simulink model "Bowwave2Drogue_v6_addControl_VR_tkTur2"  (R2013a)
settings: Solver=ode4  StartTime=0.0  StopTime=50  FixedStep=0.02  RelTol=1e-5  AbsTol=1e-4
InitFcn:
  | F16InitData_slow
values from neighbouring files (symbols this model uses):
  A_full = [ ... (first row only)    [F16InitData.m]    (also in F16InitData_slow.m)
  B_full = [ ... (first row only)    [F16InitData.m]    (also in F16InitData_slow.m)
  B_wTur = zeros(12,6)    [F16InitData.m]    (also in F16InitData_slow.m = A_full*Csta*Cb_e; F16_2003hiModelAutopilot.m = A*Csta*Cb_e)
  C_attitude = [0 0 0 1 0 0 0 0 0 0 0 0 ... (first row only)    [F16InitData.m]    (also in F16InitData_slow.m; F16_2003hiModelAutopilot.m = [zeros(3,3),eye(3),zeros(3,12)])
  C_xd_h_yd = [ ... (first row only)    [F16InitData.m]    (also in F16InitData_slow.m)
  C_xd_h_yd2m = [C_xd_h_yd2m(1,:) ... (first row only)    [F16InitData.m]    (also in F16InitData_slow.m)
  Kc = diag([0.3048,0.3048,0.3048,rad2degree,rad2degree,rad2degree,1,0.3048,rad2degree,rad2degree,rad2degree,rad2degree])    [F16InitData.m]    (also in F16InitData1.m = [1	0	0	0	0	0	0	0	0	0	0	0	0	0	0	0	0	0; F16InitData_slow.m; F16_2003hiModelAutopilot.m = [)
  Ki = [ ... (first row only)    [F16InitData.m]    (also in F16InitData_slow.m = [1.97872869	0.650510465	0; F16_2003hiModelAutopilot.m = zeros(4,3))
  Kp = [ ... (first row only)    [F16InitData.m]    (also in F16InitData_slow.m; F16_2003hiModelAutopilot.m = zeros(4,18))
  m2ft = 1/0.3048    (= 3.28083989501)    [F16InitData.m]    (also in F16InitData_slow.m; F16_2003hiModelAutopilot.m)
  q = zeros(N,1)    [hose3D_n_air_Fv_correction.m]
  trim_control = [-3.132 ... (first row only)    [F16InitData.m]    (also in F16InitData1.m = [-1.549425813; F16InitData_slow.m; F16_2003hiModelAutopilot.m = [-2.979731649)
  trim_state = [ ... (first row only)    [F16InitData.m]    (also in F16InitData1.m = [0; F16InitData_slow.m; F16_2003hiModelAutopilot.m)
  trim_thrust = 0.17766    [F16InitData.m]    (also in F16InitData1.m = -206727.459732; F16InitData_slow.m; F16NolinearModelInitialData.m = 5000; F16_2003hiModelAutopilot.m = 2279.08519955)
  X1_0 = [0 0 0 0 0 0 0 0 0 0 0 0]'    [F16InitData.m]    (also in F16InitData1.m = zeros(18,1); F16InitData_slow.m; F16_2003hiModelAutopilot.m = zeros(18,1))
undefined symbols (not defined in the file or in its folder): F, Light, MIL
libraries: simulink x5, aerolibwind2 x3, vrlib x1
settings Model: Creator=WhisPer  LastModifiedBy=Dai

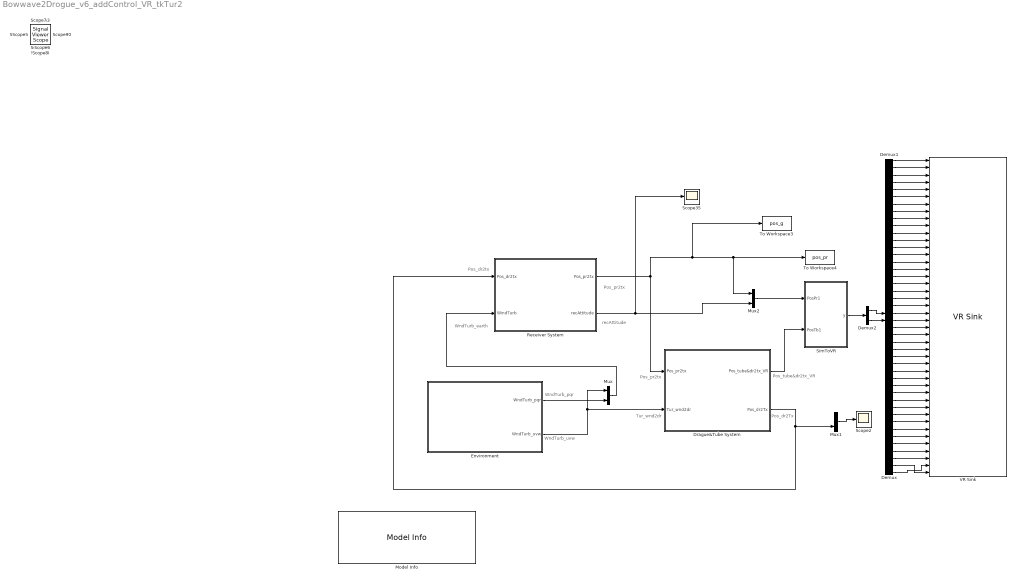
== system Bowwave2Drogue_v6_addControl_VR_tkTur2 ==
  note: recAttitude
  note: WndTurb_uvw
  note: WndTurb_pqr
  note: Pos_dr2Tx
  note: Pos_tube&dr2tx_VR
  note: Tur_wnd2dr
  note: Pos_pr2tx
  note: WndTurb_earth
  note: Pos_dr2tx
  note: Pos_pr2tx
  Demux : Demux  Outputs=22
  Demux1 : Demux  Outputs=22
  Demux2 : Demux  Outputs=[88,66]
  Drague&Tube System : Subsystem
      mask Display: image(imread('Icon\zhuitao.png'))
  Environment : Subsystem
      mask Display: image(imread('Icon\Enviroment.jpg'))
  Model Info : simulink/Model-Wide Utilities/Model Info  InitialBlockCM=None  BlockCM=None  Frame=on  DisplayStringWithTags=|  HorizontalTextAlignment=Center  LeftAlignmentValue=0.5  SourceBlockDiagram=Bowwave2Drogue_v6_addControl_VR_tkTur2  TagMaxNumber=20
      | Ppr_rc=[6.06 0.54 -0.86]
      | Pns_rc=[8.00 0.00  0.00]
      | Pfl_rc=[3.75 0.00 -0.86]
      | Pdr0_tk=[-13.549 0.00 5]
  Mux : Mux  Inputs=2
  Mux1 : Mux  Inputs=2
  Mux2 : Mux  Inputs=2
  Receiver System : Subsystem
      mask Display: image(imread('Icon\f16thumb.jpg'))
  Scope2 : Scope
      settings: YMin=-22.5  YMax=7.5  SaveName=ScopeData18
  Scope35 : Scope
      settings: YMin=-0.225  YMax=0.15  SaveName=ScopeData19
  SimToVR : MATLAB Function  TreatAsAtomicUnit=on
  To Workspace3 : ToWorkspace  VariableName=pos_g  SampleTime=-1
  To Workspace4 : ToWorkspace  VariableName=pos_pr  SampleTime=-1
  VR Sink : vrlib/VR Sink  InstantiateOnLoad=on  SampleTime=-1  ViewEnable=on  RemoteChange=off  RemoteView=off  FieldsWritten=tube1.rotation.4.1.1.double#tube1.translation.3.1.1.double#tube2.rotation.4.1.1.double#tube2.translation.3.1.1.double#tube3.rotation.4.1.1.double#tube3.translation.3.1.1.double#tube4.rotation.4.1.1.double#tube4.translation.3.1.1.double#tube5.rotation.4.1.1.double#tube5.translation.3.1.1.double#tube6.rotation.4.1.1.double#tube6.translation.3.1.1.double#tube7.rotation.4.1.1.double#tube7.translation.3.1.1.double#tube8.rotation.4.1.1.double#tube8.translation.3.1.1.double#tube9.rotation.4.1.1.double#tube9.translation.3.1.1.double#tube10.rotation.4.1.1.double#tube10.translation.3.1.1.double#tube11.rotation.4.1.1.double#tube11.translation.3.1.1.double#tube12.rotation.4.1.1.double#tube12.translation.3.1.1.double#tube13.rotation.4.1.1.double#tube13.translation.3.1.1.double#tube14.rotation.4.1.1.double#tube14.translation.3.1.1.double#tube15.rotation.4.1.1.double#tube15.translation.3.1.1.double#tube16.rotation.4.1.1.double#tube16.translation.3.1.1.double#tube17.rotation.4.1.1.double#tube17.translation.3.1.1.double#tube18.rotation.4.1.1.double#tube18.translation.3.1.1.double#tube19.rotation.4.1.1.double#tube19.translation.3.1.1.double#tube20.rotation.4.1.1.double#tube20.translation.3.1.1.double#tube21.rotation.4.1.1.double#tube21.translation.3.1.1.double#ASDD.translation.3.1.1.double#Receiver.rotation.4.1.1.double  WorldFileName=AirRefuelingTubeSim.WRL  AutoView=off  VideoDimensions=[]  AllowVariableSize=off
  Scope{,1,3,5..9,11,13,15..34} (30 alike) : SignalViewerScope  IOType=viewer  RefreshTime=0.035000
      Scope settings: SaveName=ScopeData32
      Scope1 settings: YMin=-40  YMax=15  SaveName=ScopeData33
      Scope11 settings: SaveName=ScopeData7
      Scope13 settings: SaveName=ScopeData10
      Scope15 settings: SaveName=ScopeData12
      Scope16 settings: SaveName=ScopeData13
      Scope17 settings: SaveName=ScopeData14
      Scope18 settings: SaveName=ScopeData15
      Scope19 settings: SaveName=ScopeData16
      Scope20 settings: SaveName=ScopeData17
      Scope21 settings: SaveName=ScopeData18
      Scope22 settings: SaveName=ScopeData19
      Scope23 settings: SaveName=ScopeData20
      Scope24 settings: SaveName=ScopeData21
      Scope25 settings: SaveName=ScopeData22
      Scope26 settings: SaveName=ScopeData23
      Scope27 settings: SaveName=ScopeData24
      Scope28 settings: SaveName=ScopeData25
      Scope29 settings: SaveName=ScopeData26
      Scope3 settings: TimeRange=8  YMin=-2895.619158878505  YMax=-1095.619158878505
      Scope30 settings: SaveName=ScopeData27
      Scope31 settings: SaveName=ScopeData28
      Scope32 settings: SaveName=ScopeData29
      Scope33 settings: SaveName=ScopeData30
      Scope34 settings: YMin=-0.5  YMax=0.9  SaveName=ScopeData31
      Scope5 settings: SaveName=ScopeData2
      Scope6 settings: SaveName=ScopeData3
      Scope7 settings: SaveName=ScopeData4
      Scope8 settings: SaveName=ScopeData5
      Scope9 settings: SaveName=ScopeData9
  Scope10 : SignalViewerScope  IOType=viewer  ZoomMode=yonly  RefreshTime=0.035000
      settings: SaveName=ScopeData6
  Scope12 : SignalViewerScope  IOType=viewer  ZoomMode=xonly  RefreshTime=0.035000
      settings: SaveName=ScopeData8
  Scope14 : SignalViewerScope  IOType=viewer  ZoomMode=yonly  RefreshTime=0.035000
      settings: YMin=-1  YMax=1  SaveName=ScopeData11
  Scope4 : SignalViewerScope  IOType=viewer  ZoomMode=xonly  RefreshTime=0.035000
  wires:
  Receiver System/1(Pos_pr2tx) -> Drague&Tube System/1(Pos_pr2tx), Mux2/1, To Workspace4/1, To Workspace3/1
  Demux2/1 -> Demux1/1
  Demux2/2 -> Demux/1
  SimToVR/1(y) -> Demux2/1
  Drague&Tube System/1(Pos_tube&dr2tx_VR) -> SimToVR/2(PosTb1)
  Drague&Tube System/2(Pos_dr2Tx) -> Receiver System/1(Pos_dr2tx), Mux1/2
  Mux/1 -> Receiver System/2(WindTurb)
  Environment/2(WndTurb_uvw) -> Drague&Tube System/2(Tur_wnd2dr), Mux/1
  Environment/1(WndTurb_pqr) -> Mux/2
  Mux1/1 -> Scope2/1
  Receiver System/2(recAttitude) -> Scope35/1, Mux2/2
  Mux2/1 -> SimToVR/1(PosPr1)
  Demux1/1 -> VR Sink/1
  Demux/1 -> VR Sink/2
  Demux1/2 -> VR Sink/3
  Demux/2 -> VR Sink/4
  Demux1/3 -> VR Sink/5
  Demux/3 -> VR Sink/6
  Demux1/4 -> VR Sink/7
  Demux/4 -> VR Sink/8
  Demux1/5 -> VR Sink/9
  Demux/5 -> VR Sink/10
  Demux1/6 -> VR Sink/11
  Demux/6 -> VR Sink/12
  Demux1/7 -> VR Sink/13
  Demux/7 -> VR Sink/14
  Demux1/8 -> VR Sink/15
  Demux/8 -> VR Sink/16
  Demux1/9 -> VR Sink/17
  Demux/9 -> VR Sink/18
  Demux1/10 -> VR Sink/19
  Demux/10 -> VR Sink/20
  Demux1/11 -> VR Sink/21
  Demux/11 -> VR Sink/22
  Demux1/12 -> VR Sink/23
  Demux/12 -> VR Sink/24
  Demux1/13 -> VR Sink/25
  Demux/13 -> VR Sink/26
  Demux1/14 -> VR Sink/27
  Demux/14 -> VR Sink/28
  Demux1/15 -> VR Sink/29
  Demux/15 -> VR Sink/30
  Demux1/16 -> VR Sink/31
  Demux/16 -> VR Sink/32
  Demux1/17 -> VR Sink/33
  Demux/17 -> VR Sink/34
  Demux1/18 -> VR Sink/35
  Demux/18 -> VR Sink/36
  Demux1/19 -> VR Sink/37
  Demux/19 -> VR Sink/38
  Demux1/20 -> VR Sink/39
  Demux/20 -> VR Sink/40
  Demux1/21 -> VR Sink/41
  Demux/21 -> VR Sink/42
  Demux/22 -> VR Sink/43
  Demux1/22 -> VR Sink/44

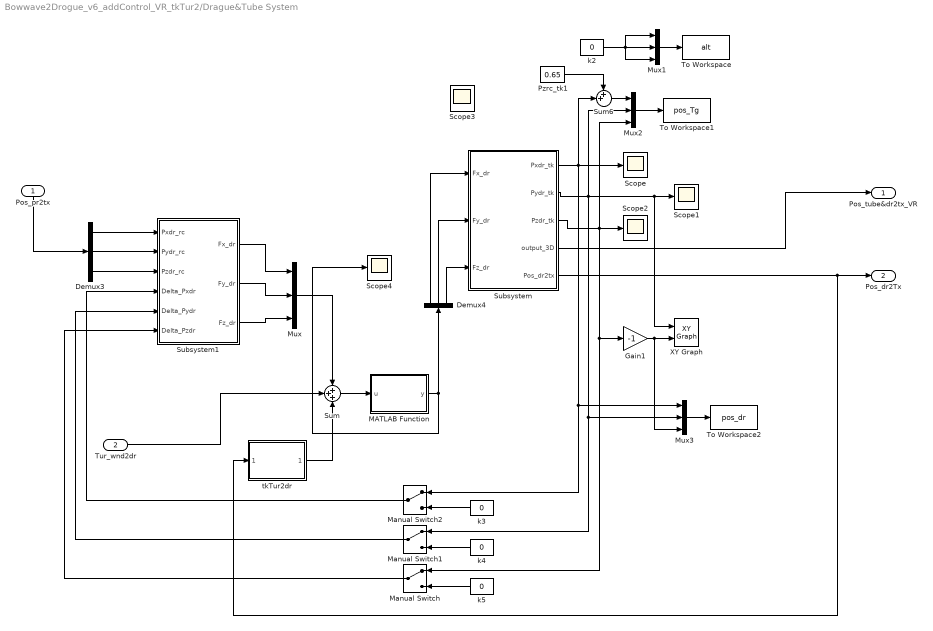
== system Bowwave2Drogue_v6_addControl_VR_tkTur2/Drague&Tube System ==
  Pos_pr2tx : Inport
  Tur_wnd2dr : Inport  Port=2
  Demux3 : Demux  Outputs=3
  Demux4 : Demux  Outputs=3
  Gain1 : Gain  Gain=-1
  MATLAB Function : MATLAB Function  TreatAsAtomicUnit=on
  Manual Switch : ManualSwitch
  Manual Switch1 : ManualSwitch
  Manual Switch2 : ManualSwitch
  Mux{,1..3} (4 alike) : Mux  Inputs=3
  Pzrc_tk1 : Constant  Value=0.65
  Scope{,1..4} (5 alike) : Scope
      Scope1 settings: YMin=-1  YMax=1
      Scope2 settings: SaveName=ScopeData2
      Scope3 settings: YMin=-15.5  YMax=-9  SaveName=ScopeData17
      Scope4 settings: TimeRange=50  YMin=-60  SaveName=ScopeData20
  Subsystem : Subsystem
  Subsystem1 : Subsystem
  Sum : Sum  Inputs=+++
  Sum6 : Sum  Inputs=++|
  To Workspace : ToWorkspace  VariableName=alt  SampleTime=-1
  To Workspace1 : ToWorkspace  VariableName=pos_Tg  SampleTime=-1
  To Workspace2 : ToWorkspace  VariableName=pos_dr  SampleTime=-1
  XY Graph : simulink/Sinks/XY Graph  xmin=-1  xmax=1  ymin=-1-4.65  ymax=1-4.65  st=-1
  k{2..5} (4 alike) : Constant  Value=0
  tkTur2dr : MATLAB Function  TreatAsAtomicUnit=on
  Pos_tube&dr2tx_VR : Outport
  Pos_dr2Tx : Outport  Port=2
  wires:
  Demux3/2 -> Subsystem1/2(Pydr_rc)
  Demux3/3 -> Subsystem1/3(Pzdr_rc)
  Subsystem/5(Pos_dr2tx) -> tkTur2dr/1(pos_dr2tk), Pos_dr2Tx/1
  Subsystem/3(Pzdr_tk) -> Manual Switch/1, Gain1/1, Mux2/3, Scope2/1
  Gain1/1 -> Mux3/3, XY Graph/2
  Subsystem/1(Pxdr_tk) -> Mux3/1, Manual Switch2/1, Scope/1, Sum6/2
  Subsystem/2(Pydr_tk) -> Mux3/2, Manual Switch1/1, Mux2/2, XY Graph/1, Scope1/1
  Manual Switch/1 -> Subsystem1/6(Delta_Pzdr)
  Mux2/1 -> To Workspace1/1
  Mux1/1 -> To Workspace/1
  Mux3/1 -> To Workspace2/1
  k3/1 -> Manual Switch2/2
  k5/1 -> Manual Switch/2
  Pzrc_tk1/1 -> Sum6/1
  k2/1 -> Mux1/3, Mux1/1, Mux1/2
  Sum6/1 -> Mux2/1
  Manual Switch2/1 -> Subsystem1/4(Delta_Pxdr)
  Manual Switch1/1 -> Subsystem1/5(Delta_Pydr)
  k4/1 -> Manual Switch1/2
  Subsystem/4(output_3D) -> Pos_tube&dr2tx_VR/1
  MATLAB Function/1(y) -> Demux4/1, Scope4/1
  Pos_pr2tx/1 -> Demux3/1
  Demux3/1 -> Subsystem1/1(Pxdr_rc)
  Subsystem1/1(Fx_dr) -> Mux/1
  Subsystem1/2(Fy_dr) -> Mux/2
  Sum/1 -> MATLAB Function/1(u)
  Mux/1 -> Sum/1
  Demux4/1 -> Subsystem/1(Fx_dr)
  Demux4/2 -> Subsystem/2(Fy_dr)
  Demux4/3 -> Subsystem/3(Fz_dr)
  Subsystem1/3(Fz_dr) -> Mux/3
  Tur_wnd2dr/1 -> Sum/2
  tkTur2dr/1(TkTur2dr) -> Sum/3

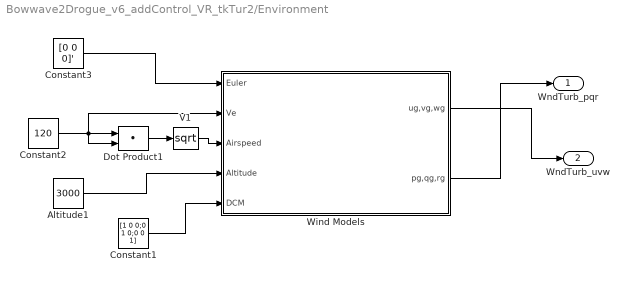
== system Bowwave2Drogue_v6_addControl_VR_tkTur2/Environment ==
  Altitude1 : Constant  Value=3000
  Constant1 : Constant  Value=[1 0 0;0 1 0;0 0 1]
  Constant2 : Constant  Value=120
  Constant3 : Constant  Value=[0 0 0]'
  Dot Product1 : DotProduct  SaturateOnIntegerOverflow=on  OutDataTypeStr=Inherit: Inherit via internal rule
  V1 : Math  Operator=sqrt  SaturateOnIntegerOverflow=on
  Wind Models : Subsystem  AncestorBlock=aeroblk_lib_HL20/HL20 Airframe/Environment Models/Wind Models
  WndTurb_pqr : Outport
  WndTurb_uvw : Outport  Port=2
  wires:
  Wind Models/2(pg,qg,rg) -> WndTurb_pqr/1
  Dot Product1/1 -> V1/1
  Constant3/1 -> Wind Models/1(Euler)
  Wind Models/1(ug,vg,wg) -> WndTurb_uvw/1
  Constant2/1 -> Wind Models/2(Ve), Dot Product1/1, Dot Product1/2
  V1/1 -> Wind Models/3(Airspeed)
  Constant1/1 -> Wind Models/5(DCM)
  Altitude1/1 -> Wind Models/4(Altitude)

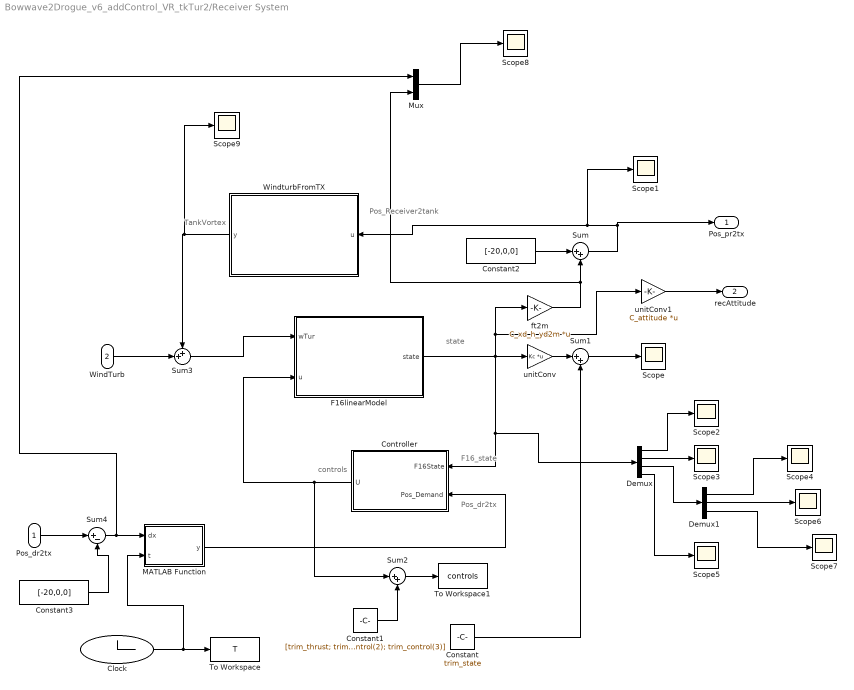
== system Bowwave2Drogue_v6_addControl_VR_tkTur2/Receiver System ==
  note: controls
  note: Pos_dr2tx
  note: F16_state
  note: TankVortex
  note: Pos_Receiver2tank
  note: state
  Pos_dr2tx : Inport
  WindTurb : Inport  Port=2
  Clock : Clock
      settings: Decimation=50
  Constant : Constant  Value=trim_state
  Constant1 : Constant  Value=[trim_thrust; trim_control(1); trim_control(2); trim_control(3)]
  Constant2 : Constant  Value=[-20,0,0]
  Constant3 : Constant  Value=[-20,0,0]
  Controller : Subsystem
      mask Display: image(imread('Icon\F16_Pilot.jpg'))
  Demux : Demux
  Demux1 : Demux  Outputs=3
  F16linearModel : Subsystem
      mask Display: image(imread('Icon\fighter_f16.jpg'))
  MATLAB Function : MATLAB Function  TreatAsAtomicUnit=on
  Mux : Mux  Inputs=2
  Scope{,1..9} (10 alike) : Scope
      Scope settings: YMin=-250  YMax=3000  SaveName=ScopeData5
      Scope1 settings: YMin=-27.5  YMax=7.5  SaveName=ScopeData7
      Scope2 settings: TimeRange=30  YMin=-90  YMax=20  SaveName=ScopeData10
      Scope3 settings: TimeRange=30  YMin=-0.00025  YMax=0.0002  SaveName=ScopeData11
      Scope4 settings: TimeRange=30  YMin=-75  YMax=225  SaveName=ScopeData12
      Scope5 settings: TimeRange=30  YMin=-9e-09  YMax=2e-09  SaveName=ScopeData13
      Scope6 settings: TimeRange=30  YMin=-0.00025  YMax=0.0002  SaveName=ScopeData14
      Scope7 settings: TimeRange=30  YMin=-0.00025  YMax=0.0002  SaveName=ScopeData15
      Scope8 settings: YMin=-2  YMax=7.5  SaveName=ScopeData16
      Scope9 settings: YMin=-0.25  YMax=4.5  SaveName=ScopeData21
  Sum : Sum  Inputs=|++
  Sum1 : Sum  Inputs=|++  SaturateOnIntegerOverflow=on  InputSameDT=on  OutDataTypeStr=Inherit: Same as first input
  Sum2 : Sum  Inputs=|++  SaturateOnIntegerOverflow=on  InputSameDT=on  OutDataTypeStr=Inherit: Same as first input
  Sum3 : Sum  Inputs=++|
  Sum4 : Sum  Inputs=|+-
  To Workspace : ToWorkspace  VariableName=T  SampleTime=-1
      settings: Decimation=100
  To Workspace1 : ToWorkspace  VariableName=controls  SampleTime=-1
      settings: Decimation=100
  WindturbFromTX : MATLAB Function  TreatAsAtomicUnit=on
  ft2m : Gain  Gain=C_xd_h_yd2m  Multiplication=Matrix(K*u) (u vector)
  unitConv : Gain  Gain=Kc  Multiplication=Matrix(K*u) (u vector)
  unitConv1 : Gain  Gain=C_attitude  Multiplication=Matrix(K*u) (u vector)
  Pos_pr2tx : Outport
  recAttitude : Outport  Port=2
  wires:
  Controller/1(U) -> Sum2/1, F16linearModel/2(u)
  Clock/1 -> MATLAB Function/2(t), To Workspace/1
  F16linearModel/1(state) -> ft2m/1, unitConv1/1, Demux/1, Controller/1(F16State), unitConv/1
  Constant1/1 -> Sum2/2
  Sum2/1 -> To Workspace1/1
  Constant/1 -> Sum1/2
  unitConv/1 -> Sum1/1
  WindTurb/1 -> Sum3/2
  Sum1/1 -> Scope/1
  MATLAB Function/1(y) -> Controller/2(Pos_Demand)
  Demux/1 -> Scope2/1
  Demux/2 -> Scope3/1
  Demux/3 -> Demux1/1
  Demux/4 -> Scope5/1
  Sum3/1 -> F16linearModel/1(wTur)
  Demux1/1 -> Scope4/1
  Demux1/2 -> Scope6/1
  Demux1/3 -> Scope7/1
  ft2m/1 -> Mux/2, Sum/2
  Constant2/1 -> Sum/1
  Sum/1 -> Scope1/1, WindturbFromTX/1(u), Pos_pr2tx/1
  Pos_dr2tx/1 -> Sum4/1
  Sum4/1 -> Mux/1, MATLAB Function/1(dx)
  Constant3/1 -> Sum4/2
  Mux/1 -> Scope8/1
  unitConv1/1 -> recAttitude/1
  WindturbFromTX/1(y) -> Scope9/1, Sum3/1

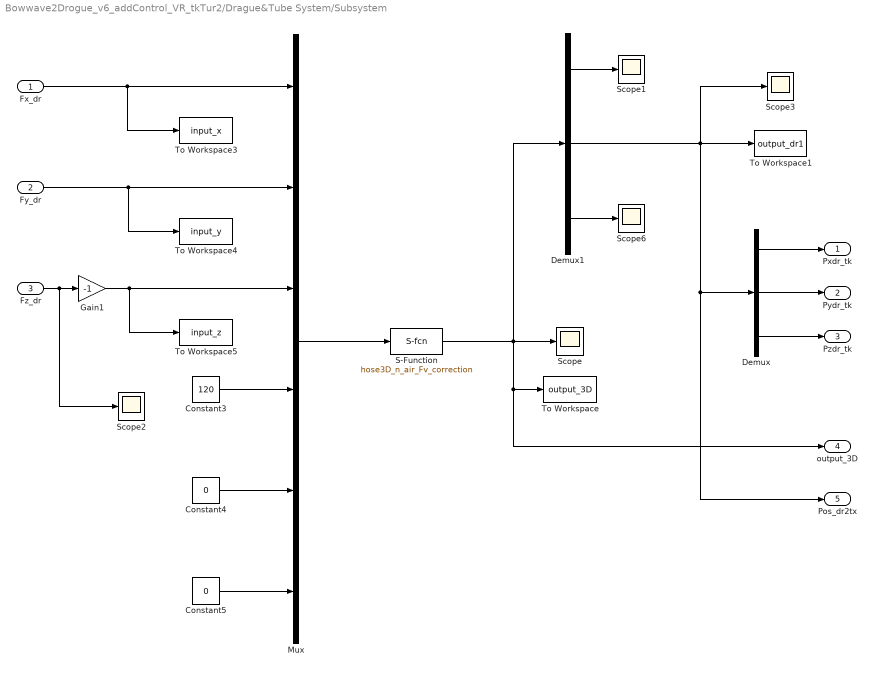
== system Bowwave2Drogue_v6_addControl_VR_tkTur2/Drague&Tube System/Subsystem ==
  Fx_dr : Inport
  Fy_dr : Inport  Port=2
  Fz_dr : Inport  Port=3
  Constant3 : Constant  Value=120
  Constant4 : Constant  Value=0
  Constant5 : Constant  Value=0
  Demux : Demux  Outputs=3
  Demux1 : Demux  Outputs=[57,3,40]
  Gain1 : Gain  Gain=-1
  Mux : Mux  Inputs=6
  S-Function : S-Function  FunctionName=hose3D_n_air_Fv_correction  EnableBusSupport=off
  Scope{,1..3,6} (5 alike) : Scope
      Scope settings: YMin=-14  YMax=1  SaveName=ScopeData4
      Scope1 settings: YMin=-14  YMax=1  SaveName=ScopeData3
      Scope2 settings: YMin=-65  YMax=0  SaveName=ScopeData8
      Scope3 settings: YMin=1025  YMax=1350  SaveName=ScopeData6
      Scope6 settings: YMin=-14  YMax=1  SaveName=ScopeData9
  To Workspace : ToWorkspace  VariableName=output_3D  SampleTime=-1
  To Workspace1 : ToWorkspace  VariableName=output_dr1  SampleTime=-1
  To Workspace3 : ToWorkspace  VariableName=input_x  SampleTime=-1
  To Workspace4 : ToWorkspace  VariableName=input_y  SampleTime=-1
  To Workspace5 : ToWorkspace  VariableName=input_z  SampleTime=-1
  Pxdr_tk : Outport
  Pydr_tk : Outport  Port=2
  Pzdr_tk : Outport  Port=3
  output_3D : Outport  Port=4
  Pos_dr2tx : Outport  Port=5
  wires:
  Mux/1 -> S-Function/1
  Constant3/1 -> Mux/4
  Constant4/1 -> Mux/5
  Constant5/1 -> Mux/6
  Fy_dr/1 -> Mux/2, To Workspace4/1
  Fz_dr/1 -> Scope2/1, Gain1/1
  Fx_dr/1 -> To Workspace3/1, Mux/1
  Demux1/1 -> Scope1/1
  Demux1/3 -> Scope6/1
  Demux1/2 -> Pos_dr2tx/1, Demux/1, To Workspace1/1, Scope3/1
  Demux/1 -> Pxdr_tk/1
  Demux/2 -> Pydr_tk/1
  Demux/3 -> Pzdr_tk/1
  Gain1/1 -> Mux/3, To Workspace5/1
  S-Function/1 -> Demux1/1, Scope/1, output_3D/1, To Workspace/1

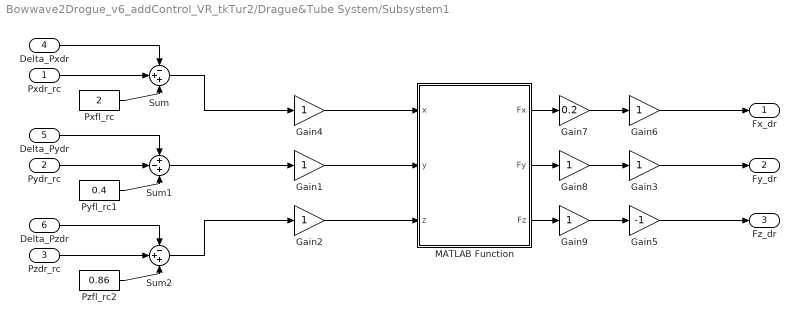
== system Bowwave2Drogue_v6_addControl_VR_tkTur2/Drague&Tube System/Subsystem1 ==
  Pxdr_rc : Inport
  Pydr_rc : Inport  Port=2
  Pzdr_rc : Inport  Port=3
  Delta_Pxdr : Inport  Port=4
  Delta_Pydr : Inport  Port=5
  Delta_Pzdr : Inport  Port=6
  Gain{1..4,6,8..9} (7 alike) : Gain
  Gain5 : Gain  Gain=-1
  Gain7 : Gain  Gain=0.2
  MATLAB Function : MATLAB Function  TreatAsAtomicUnit=on
  Pxfl_rc : Constant  Value=2
  Pyfl_rc1 : Constant  Value=0.4
  Pzfl_rc2 : Constant  Value=0.86
  Sum : Sum  Inputs=-++
  Sum1 : Sum  Inputs=+-+
  Sum2 : Sum  Inputs=-++
  Fx_dr : Outport
  Fy_dr : Outport  Port=2
  Fz_dr : Outport  Port=3
  wires:
  Sum/1 -> Gain4/1
  Sum1/1 -> Gain1/1
  Sum2/1 -> Gain2/1
  MATLAB Function/1(Fx) -> Gain7/1
  MATLAB Function/2(Fy) -> Gain8/1
  Pxdr_rc/1 -> Sum/2
  Pxfl_rc/1 -> Sum/3
  Delta_Pxdr/1 -> Sum/1
  Pydr_rc/1 -> Sum1/2
  Delta_Pydr/1 -> Sum1/1
  Pyfl_rc1/1 -> Sum1/3
  Pzdr_rc/1 -> Sum2/2
  Pzfl_rc2/1 -> Sum2/3
  Delta_Pzdr/1 -> Sum2/1
  Gain4/1 -> MATLAB Function/1(x)
  Gain1/1 -> MATLAB Function/2(y)
  Gain2/1 -> MATLAB Function/3(z)
  Gain3/1 -> Fy_dr/1
  Gain5/1 -> Fz_dr/1
  Gain6/1 -> Fx_dr/1
  MATLAB Function/3(Fz) -> Gain9/1
  Gain7/1 -> Gain6/1
  Gain8/1 -> Gain3/1
  Gain9/1 -> Gain5/1

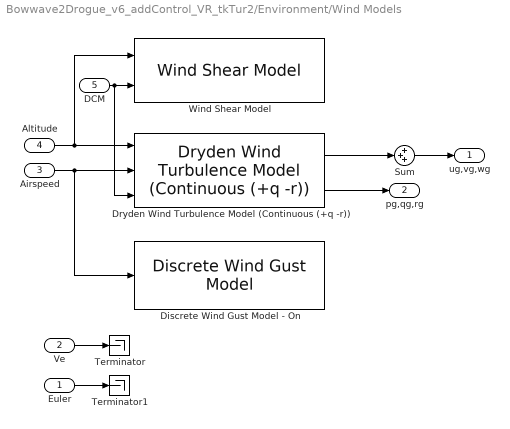
== system Bowwave2Drogue_v6_addControl_VR_tkTur2/Environment/Wind Models ==
  Euler : Inport
  Ve : Inport  Port=2
  Airspeed : Inport  Port=3
  Altitude : Inport  Port=4
  DCM : Inport  Port=5
  Discrete Wind Gust Model - On : aerolibwind2/Discrete Wind Gust Model  units=Metric (MKS)  Gx=on  Gy=on  Gz=on  t_0=20  d_m=[120 120 80]  v_m=[3.5 3.0 3.0]
  Dryden Wind Turbulence Model (Continuous (+q -r)) : aerolibwind2/Dryden Wind Turbulence Model  (Continuous (+q -r))  units=Metric (MKS)  spec=MIL-F-8785C  model=Continuous Dryden (+q -r)  W20=0  Wdeg=0  TurbProb=10^-2 - Light  L_high=6000  Wingspan=4  ts=0.02  Seed=1+fix(3650*rand(1,4))  T_on=on
  Sum : Sum  Inputs=+++  SaturateOnIntegerOverflow=on  InputSameDT=on  OutDataTypeStr=Inherit: Same as first input
  Terminator : Terminator
  Terminator1 : Terminator
  Wind Shear Model : aerolibwind2/Wind Shear Model  units=Metric (MKS)  phase=Category C - Terminal Flight Phase  W_20=1  Wdeg=0
  ug,vg,wg : Outport
  pg,qg,rg : Outport  Port=2
  wires:
  Euler/1 -> Terminator1/1
  Ve/1 -> Terminator/1
  Sum/1 -> ug,vg,wg/1
  DCM/1 -> Dryden Wind Turbulence Model (Continuous (+q -r))/3, Wind Shear Model/2
  Airspeed/1 -> Dryden Wind Turbulence Model (Continuous (+q -r))/2, Discrete Wind Gust Model - On/1
  Dryden Wind Turbulence Model (Continuous (+q -r))/2 -> pg,qg,rg/1
  Altitude/1 -> Dryden Wind Turbulence Model (Continuous (+q -r))/1, Wind Shear Model/1
  Dryden Wind Turbulence Model (Continuous (+q -r))/1 -> Sum/2

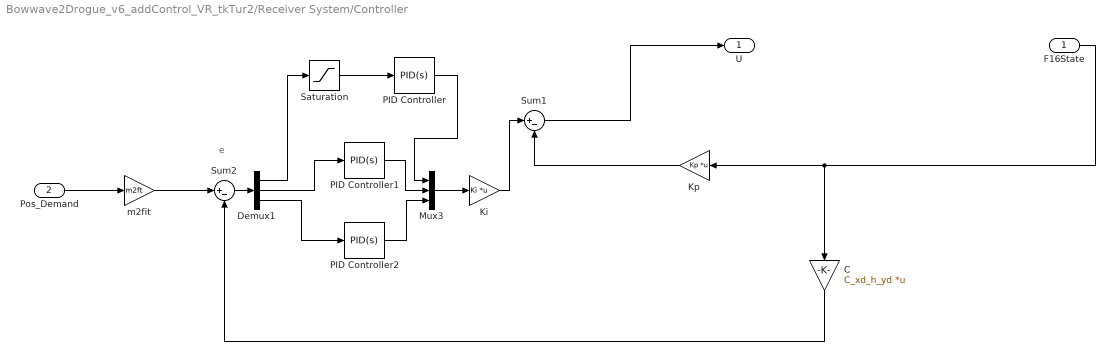
== system Bowwave2Drogue_v6_addControl_VR_tkTur2/Receiver System/Controller ==
  note: e
  F16State : Inport
  Pos_Demand : Inport  Port=2
  C : Gain  Gain=C_xd_h_yd  Multiplication=Matrix(K*u) (u vector)
  Demux1 : Demux  Outputs=3
  Ki : Gain  Gain=Ki  Multiplication=Matrix(K*u) (u vector)
  Kp : Gain  Gain=Kp  Multiplication=Matrix(K*u) (u vector)
  Mux3 : Mux  Inputs=3
  PID Controller : simulink/Continuous/PID Controller  Controller=PID  TimeDomain=Continuous-time  SampleTime=1  IntegratorMethod=Forward Euler  FilterMethod=Forward Euler  Form=Parallel  P=0  I=1.2  D=0  N=100  InitialConditionSource=internal  InitialConditionForIntegrator=0  InitialConditionForFilter=0  ExternalReset=none  LimitOutput=off  UpperSaturationLimit=inf  LowerSaturationLimit=-inf  LinearizeAsGain=on  AntiWindupMode=none  Kb=1  TrackingMode=off  Kt=1  PParamMin=[]  PParamMax=[]  IParamMin=[]  IParamMax=[]  DParamMin=[]  DParamMax=[]  NParamMin=[]  NParamMax=[]  KbParamMin=[]  KbParamMax=[]  KtParamMin=[]  KtParamMax=[]  POutMin=[]  POutMax=[]  IOutMin=[]  IOutMax=[]  DOutMin=[]  DOutMax=[]  NOutMin=[]  NOutMax=[]  KbOutMin=[]  KbOutMax=[]  KtOutMin=[]  KtOutMax=[]  IntegratorOutMin=[]  IntegratorOutMax=[]  FilterOutMin=[]  FilterOutMax=[]  SumOutMin=[]  SumOutMax=[]  SumI1OutMin=[]  SumI1OutMax=[]  SumI2OutMin=[]  SumI2OutMax=[]  SumI3OutMin=[]  SumI3OutMax=[]  SumDOutMin=[]  SumDOutMax=[]  SaturationOutMin=[]  SaturationOutMax=[]  IntegratorContinuousStateAttributes=''  IntegratorStateMustResolveToSignalObject=off  IntegratorRTWStateStorageClass=Auto  FilterContinuousStateAttributes=''  FilterStateMustResolveToSignalObject=off  FilterRTWStateStorageClass=Auto
  PID Controller1 : simulink/Continuous/PID Controller  Controller=PID  TimeDomain=Continuous-time  SampleTime=1  IntegratorMethod=Forward Euler  FilterMethod=Forward Euler  Form=Parallel  P=0  I=1.5  D=0  N=100  InitialConditionSource=internal  InitialConditionForIntegrator=0  InitialConditionForFilter=0  ExternalReset=none  LimitOutput=off  UpperSaturationLimit=inf  LowerSaturationLimit=-inf  LinearizeAsGain=on  AntiWindupMode=none  Kb=1  TrackingMode=off  Kt=1  PParamMin=[]  PParamMax=[]  IParamMin=[]  IParamMax=[]  DParamMin=[]  DParamMax=[]  NParamMin=[]  NParamMax=[]  KbParamMin=[]  KbParamMax=[]  KtParamMin=[]  KtParamMax=[]  POutMin=[]  POutMax=[]  IOutMin=[]  IOutMax=[]  DOutMin=[]  DOutMax=[]  NOutMin=[]  NOutMax=[]  KbOutMin=[]  KbOutMax=[]  KtOutMin=[]  KtOutMax=[]  IntegratorOutMin=[]  IntegratorOutMax=[]  FilterOutMin=[]  FilterOutMax=[]  SumOutMin=[]  SumOutMax=[]  SumI1OutMin=[]  SumI1OutMax=[]  SumI2OutMin=[]  SumI2OutMax=[]  SumI3OutMin=[]  SumI3OutMax=[]  SumDOutMin=[]  SumDOutMax=[]  SaturationOutMin=[]  SaturationOutMax=[]  IntegratorContinuousStateAttributes=''  IntegratorStateMustResolveToSignalObject=off  IntegratorRTWStateStorageClass=Auto  FilterContinuousStateAttributes=''  FilterStateMustResolveToSignalObject=off  FilterRTWStateStorageClass=Auto
  PID Controller2 : simulink/Continuous/PID Controller  Controller=PID  TimeDomain=Continuous-time  SampleTime=1  IntegratorMethod=Forward Euler  FilterMethod=Forward Euler  Form=Parallel  P=0  I=1  D=0  N=100  InitialConditionSource=internal  InitialConditionForIntegrator=0  InitialConditionForFilter=0  ExternalReset=none  LimitOutput=off  UpperSaturationLimit=inf  LowerSaturationLimit=-inf  LinearizeAsGain=on  AntiWindupMode=none  Kb=1  TrackingMode=off  Kt=1  PParamMin=[]  PParamMax=[]  IParamMin=[]  IParamMax=[]  DParamMin=[]  DParamMax=[]  NParamMin=[]  NParamMax=[]  KbParamMin=[]  KbParamMax=[]  KtParamMin=[]  KtParamMax=[]  POutMin=[]  POutMax=[]  IOutMin=[]  IOutMax=[]  DOutMin=[]  DOutMax=[]  NOutMin=[]  NOutMax=[]  KbOutMin=[]  KbOutMax=[]  KtOutMin=[]  KtOutMax=[]  IntegratorOutMin=[]  IntegratorOutMax=[]  FilterOutMin=[]  FilterOutMax=[]  SumOutMin=[]  SumOutMax=[]  SumI1OutMin=[]  SumI1OutMax=[]  SumI2OutMin=[]  SumI2OutMax=[]  SumI3OutMin=[]  SumI3OutMax=[]  SumDOutMin=[]  SumDOutMax=[]  SaturationOutMin=[]  SaturationOutMax=[]  IntegratorContinuousStateAttributes=''  IntegratorStateMustResolveToSignalObject=off  IntegratorRTWStateStorageClass=Auto  FilterContinuousStateAttributes=''  FilterStateMustResolveToSignalObject=off  FilterRTWStateStorageClass=Auto
  Saturation : Saturate  UpperLimit=8  LowerLimit=-8
  Sum1 : Sum  Inputs=|+-
  Sum2 : Sum  Inputs=|+-
  m2fit : Gain  Gain=m2ft
  U : Outport
  wires:
  Sum2/1 -> Demux1/1
  Kp/1 -> Sum1/2
  Ki/1 -> Sum1/1
  C/1 -> Sum2/2
  Pos_Demand/1 -> m2fit/1
  Mux3/1 -> Ki/1
  Demux1/2 -> PID Controller1/1
  F16State/1 -> Kp/1, C/1
  PID Controller1/1 -> Mux3/2
  PID Controller/1 -> Mux3/1
  Demux1/3 -> PID Controller2/1
  PID Controller2/1 -> Mux3/3
  m2fit/1 -> Sum2/1
  Demux1/1 -> Saturation/1
  Saturation/1 -> PID Controller/1
  Sum1/1 -> U/1

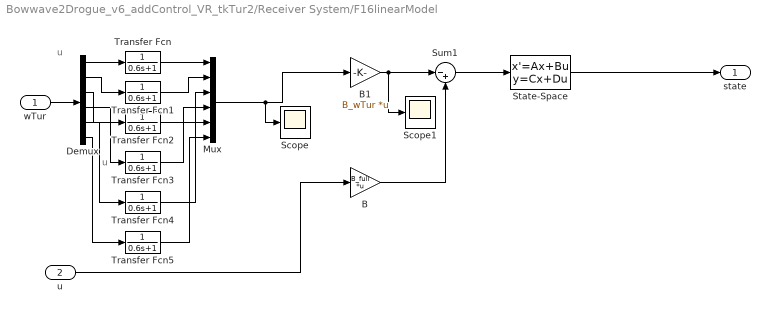
== system Bowwave2Drogue_v6_addControl_VR_tkTur2/Receiver System/F16linearModel ==
  note: u
  note: u
  wTur : Inport
  u : Inport  Port=2
  B : Gain  Gain=B_full  Multiplication=Matrix(K*u) (u vector)
  B1 : Gain  Gain=B_wTur  Multiplication=Matrix(K*u) (u vector)
  Demux : Demux  Outputs=6
  Mux : Mux  Inputs=6
  Scope : Scope
      settings: YMin=-0.5  YMax=4.75  SaveName=ScopeData22
  Scope1 : Scope
      settings: YMin=-17.5  YMax=2.5  SaveName=ScopeData23
  State-Space : StateSpace  A=A_full  B=eye(12)  C=eye(12)  D=zeros(12,12)  X0=X1_0
  Sum1 : Sum  Inputs=|-+
  Transfer Fcn{,1..5} (6 alike) : TransferFcn  Denominator=[0.6 1]
  state : Outport
  wires:
  u/1 -> B/1
  B/1 -> Sum1/2
  Sum1/1 -> State-Space/1
  B1/1 -> Scope1/1, Sum1/1
  State-Space/1 -> state/1
  wTur/1 -> Demux/1
  Demux/1 -> Transfer Fcn/1
  Transfer Fcn/1 -> Mux/1
  Demux/2 -> Transfer Fcn1/1
  Demux/3 -> Transfer Fcn2/1
  Demux/4 -> Transfer Fcn3/1
  Demux/5 -> Transfer Fcn4/1
  Demux/6 -> Transfer Fcn5/1
  Transfer Fcn1/1 -> Mux/2
  Transfer Fcn2/1 -> Mux/3
  Transfer Fcn3/1 -> Mux/4
  Transfer Fcn4/1 -> Mux/5
  Transfer Fcn5/1 -> Mux/6
  Mux/1 -> Scope/1, B1/1

== matlab function Bowwave2Drogue_v6_addControl_VR_tkTur2/Receiver System/MATLAB Function ==
  data: dx input; y output; t input
function y = fcn(dx,t)
%#codegen

dx=[dx(1);-dx(3);dx(2)];



% if t<5
%     y=[2;-10;-4];
% elseif t<10
%     y=[1;10;4];
% elseif t<20
%     y=[4;-10;-4];
% elseif t<40

if t<10
    y=[-1;-6;-2];
elseif t<25
     y=[-1;dx(2);dx(3)];    
else
    
    y=dx;
end

== matlab function Bowwave2Drogue_v6_addControl_VR_tkTur2/Drague&Tube System/Subsystem1/MATLAB Function ==
  data: x input; Fx output; y input; z input; Fy output; Fz output
function [Fx,Fy,Fz] = F_rc2dr(x,y,z)

% Fz = 229.5*(1-0.2122*x)*exp(-y^2/0.5341)*exp(-z/0.7166)*(0.5-1/pi*atan(1000*(x-4.71)));
% Fy = 330.9*(1-0.2181*x)*(y*exp(-y^2/0.878))*exp(-z/0.5684)*(0.5-1/pi*atan(1000*(x-4.615)));
% Fx = 121.2224*(1-0.3918*(x-3.9316)^2)*exp(-y^2/2.226)*exp(-z/1.673)*(0.5-1/pi*atan(1000*(x-5.55)))...
%                     +519*(1-0.325*x)*exp(-y^2/0.5599)*exp(-z/0.8122)*(0.5-1/pi*atan(1000*(x-3.048)));


% 
% if x > 1/0.2161
%     Fz = 0;
% else
%     Fz = 174.0219*(1-0.2161*x)*exp(-y^2/0.5862)*exp(-z/0.6364);
% end
% 
% if x > 1/0.2128
%     Fy = 0;
% else
%     Fy = 223.4144*(1-0.2128*x)*(y*exp(-y^2/0.8480))*exp(-z/0.6874);
% end
% 
% if x > sqrt(1/0.3774)+3.9471
%     Fx = 0;
% elseif x > 1/0.3149
%     Fx = 92.0795*(1-0.3774*(x-3.9471)^2)*exp(-y^2/2.6073)*exp(-z/1.5244);
% else
%     Fx = 92.0795*(1-0.3774*(x-3.9471)^2)*exp(-y^2/2.6073)*exp(-z/1.5244)...
%                  + 338.6175*(1-0.3149*x)*exp(-y^2/0.4435)*exp(-z/1.0890);
% end



V0 = 120;
xc = 0.01;
yc = 0;
zc = 0;

xr=2.235;
yr=0.4839;


theta_x = 0.22288;

if x<=xc
    Fx = -V0*exp(-2.5*(sqrt((x-xc)^2+(y-yc)^2+(z-zc)^2)+0.75541));
elseif x<=xc+2
    Fx = -V0*exp(-2.5*(sqrt((x-xc)^2/0.85+(y-yc)^2+(z-zc)^2)+0.75541))+V0*sin(theta_x)^2*exp(-5*abs(abs(sqrt(y^2+z^2)/x)-tan(theta_x)))-V0*exp(-2.6*(sqrt((x-xr)^2/2+(y-yr)^2+(z-zc)^2)+1.1));
else
    Fx=-V0*exp(-2.5*(sqrt((x-xc)^2/0.85+(y-yc)^2+(z-zc)^2)+0.75541))+V0*sin(theta_x)^2*exp(-5*abs(abs(sqrt(y^2+z^2)/x)-tan(theta_x)))-V0*exp(-2.6*(sqrt((x-xr)^2/2+(y-yr)^2+(z-zc)^2)+1.1));
    if abs(Fx)>100
        Fx=100*sign(Fx);
    end
end




deltaTheta = 0;

tt1 = 0.22288;
tt2 = 0;
theta1 = tt1 - deltaTheta;
theta2 = tt2 - deltaTheta;


kc = tan((theta1+theta2)/2.5);
xxc = x;
yyc = kc*xxc;

r = sqrt((y-yyc)^2+z^2);

if (y-yyc)>=0
    beta1 = atan(z/(y-yyc));
else
     beta1 = atan(z/(y-yyc))+pi;
end

theta = theta1*cos(beta1/2);

if x>=0
    alpha = atan(r/x);
else
    alpha = atan(r/x)+pi;
end

if abs(r)<0.0001
    Fz=0;
    Fy=0;
else
    f =0.6*V0*sin(theta)*cos(theta)*exp(-1.5*(1+r/1.5)*abs(alpha-theta));
    Fy=(y-yyc)/r*f;
    Fz=z/r*f;
end

== matlab function Bowwave2Drogue_v6_addControl_VR_tkTur2/SimToVR ==
  data: y output; PosPr1 input; PosTb1 input
function y = SimToVR(PosPr1,PosTb1)
%#codegen

%%函数名：SimToVR
%%用途  ：将软管锥套坐标输出转换为VR输入
%%输入  ：PosPr - 受油机椎管坐标， PlsTb - 软管坐标数据
%%输出  ：VrPos - 软管和受油机VR位置，VrAngle - 旋转角度输出
%%作者  ：戴训华
%%时间  ：2014/3/19

PosPr = PosPr1(1:3);
AttitudeRecei = [PosPr1(6);-PosPr1(5);PosPr1(4)];

PosTb = PosTb1(1:60);

VrAngle = zeros(22*4,1);
VrPos = zeros(22*3,1);


for j = 1:21                        %前20为软管坐标数据，后1为软管平滑过渡处理
    if j == 1
        pX = [0, 0, 0]';            %软管起点
        pY = PosTb(3*j-2:3*j);      %软杆终点
    elseif j == 21                  %多加一段杆，做过渡
        pX = PosTb(3*j-5:3*j-3);
        pY = [PosTb(3*j-5)-0.7163*cos(8/180*pi),PosTb(3*j-4),PosTb(3*j-3)+0.7163*sin(8/180*pi)]';
    else
        pX = PosTb(3*j-5:3*j-3);
        pY = PosTb(3*j-2:3*j); 
    end
    
    pZ = (pX + pY)/2;               %中点坐标
    pZ = pZ * 8/3;                  %到VR中比例的缩放

    vAxis = [0,0,-1]';               %水平轴
    vTb = pY - pX;                  %杆的方向
    
    axis1 = null([vAxis';vTb']);%获取垂直向量
    vRot = axis1(:,1)';             %得到旋转轴
    
    if vRot(2) < 0
        vRot = -vRot;
    end
    
    VrAngle(4*j-3:4*j-1) = [vRot(1),vRot(3),vRot(2)]';
    VrAngle(4*j) = acos(vAxis'*vTb / sqrt(vAxis'*vAxis * vTb'*vTb));
    
    VrPos(3*j-2:3*j) = [pZ(1),-pZ(3),pZ(2)]';
end
%y = u;
VrAngle(85:88)=[sin(AttitudeRecei(1));sin(AttitudeRecei(2));sin(AttitudeRecei(3));norm(AttitudeRecei)];
pZ = PosPr+[0 -0.1 -0.7]';
pZ = pZ * 8/3;
VrPos(3*22-2:3*22) = [pZ(1),-pZ(3),pZ(2)]';

y = [VrAngle;VrPos];

== matlab function Bowwave2Drogue_v6_addControl_VR_tkTur2/Drague&Tube System/MATLAB Function ==
  data: u input; y output
function y = Dr_wnd2Frc(u)
%#codegen

Ve=120;
rho = 0.98;
Q=0.5*rho*Ve^2;
S=0.38;
CD=0.81*0.5;

uu=u(1);
vv=u(2);
ww=u(3);

%beta = acos(sqrt(vv^2+ww^2)/abs(uu));
%theta = atan(ww/vv);

C_beta = 0.3979;

yx=rho*S*CD*Ve*uu;
yy=Q*S*C_beta*vv/Ve;
yz=Q*S*C_beta*ww/Ve;


y = [yx,yy,yz]';

== matlab function Bowwave2Drogue_v6_addControl_VR_tkTur2/Receiver System/WindturbFromTX ==
  data: u input; y output
function y = WindTurFromTank(u)
%#codegen

%横纵向气流角速度等下计算长度
c_lat=5;
c_lon=5;

%两端参考点
u1 = u+[0 ,c_lat ,0]';
u2 = u+[0 ,-c_lat, 0]';

yy1 = TankerVortexWindField(u1);
yy2 = TankerVortexWindField(u2);

%计算x轴向滚转角速度
yp = (yy1(3) - yy2(3))/2/c_lat;

u3=u+[c_lon, 0,0]';
u4=u+[-c_lon ,0,0]';
yy3 = TankerVortexWindField(u3);
yy4 = TankerVortexWindField(u4);

%俯仰角速度计算
yq = -(yy3(3) - yy4(3))/2/c_lon;

%偏航角速度设为0
yr = 0;

%质心处风场计算
y_uvw = TankerVortexWindField(u);


y = [y_uvw(1);y_uvw(2);y_uvw(3);-yp;-yq;-yr];

== matlab function Bowwave2Drogue_v6_addControl_VR_tkTur2/Drague&Tube System/tkTur2dr ==
  data: pos_dr2tk input; TkTur2dr output
function TkTur2dr = fcn(pos_dr2tk)
%#codegen

TkTur2dr = TankerVortexWindField(pos_dr2tk);
